simulink model "system1"  (R2020a)
settings: Solver=ode45  StartTime=0.0  StopTime=1  RelTol=1e-3
libraries: powerlib x28
settings Model: Creator=srish  LastModifiedBy=srishtik
settings DataIOCC: LimitDataPoints=on  SaveFormat=Array
settings OptimizationCC: BooleanDataType=off  LifeSpan=inf
settings DebuggingCC: ReadBeforeWriteMsg=DisableAll  WriteAfterWriteMsg=DisableAll  WriteAfterReadMsg=DisableAll  SaveWithParameterizedLinksMsg=none  UnderspecifiedInitializationDetection=Classic  MergeDetectMultiDrivingBlocksExec=none  MultiTaskDSMMsg=none  SFUnexpectedBacktrackingDiag=warning  SFNoUnconditionalDefaultTransitionDiag=warning  SFExecutionAtInitializationDiag=none  ArithmeticOperatorsInVariantConditions=warning
settings HardwareCC: ProdBitPerPointer=32  ProdBitPerSizeT=32  ProdBitPerPtrDiffT=32  ProdLargestAtomicFloat=None  ProdIntDivRoundTo=Undefined  ProdEndianess=Unspecified  ProdWordSize=32  ProdHWDeviceType=32-bit Generic  TargetUnknown=on
settings ModelReferenceCC: UpdateModelReferenceTargets=IfOutOfDate  PropagateSignalLabelsOutOfModel=off
settings SFSimCC: SFSimEcho=off  SimUseLocalCustomCode=off  CustomCodeUndefinedFunction=UseInterfaceOnly
settings RTWCC: RTWUseLocalCustomCode=off
settings CodeAppCC: StateflowObjectComments=on
settings GRTTargetCC: TargetLangStandard=C89/C90 (ANSI)
settings ConfigComp: CovMetricSettings=dw  CovHtmlReporting=on  CovSaveCumulativeToWorkspaceVar=on  CovSaveSingleToWorkspaceVar=on  CovExternalEMLEnable=off  CovSFcnEnable=off
settings SimscapeCC: SimscapeNormalizeSystem=off

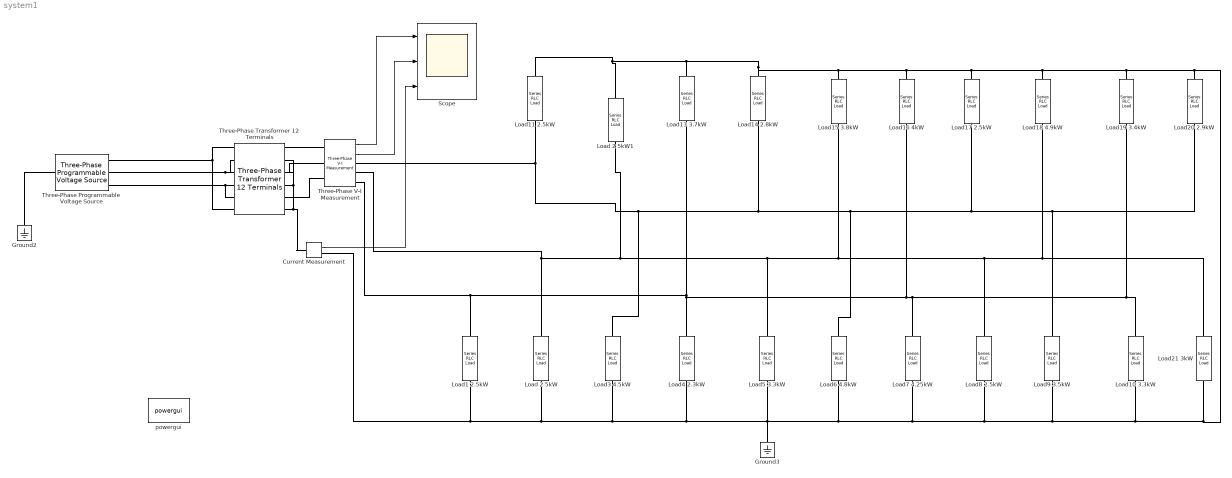
== system system1 ==
  " Load1 2.5kW" : powerlib/Elements/Series RLC Load  LConnTagsString=a  RConnTagsString=__new0  NominalVoltage=254  NominalFrequency=50  ActivePower=2500  InductivePower=1550  CapacitivePower=0  Setx0=off  InitialVoltage=0  SetiL0=off  InitialCurrent=0  Measurements=None  LoadType=constant Z
  " Load10 3.3kW " : powerlib/Elements/Series RLC Load  LConnTagsString=a  RConnTagsString=__new0  NominalVoltage=254  NominalFrequency=50  ActivePower=3300  InductivePower=2046  CapacitivePower=0  Setx0=off  InitialVoltage=0  SetiL0=off  InitialCurrent=0  Measurements=None  LoadType=constant Z
  " Load11 2.5kW" : powerlib/Elements/Series RLC Load  LConnTagsString=a  RConnTagsString=__new0  NominalVoltage=254  NominalFrequency=50  ActivePower=2500  InductivePower=1550  CapacitivePower=0  Setx0=off  InitialVoltage=0  SetiL0=off  InitialCurrent=0  Measurements=None  LoadType=constant Z
  " Load13 3.7kW" : powerlib/Elements/Series RLC Load  LConnTagsString=a  RConnTagsString=__new0  NominalVoltage=254  NominalFrequency=50  ActivePower=3700  InductivePower=2294  CapacitivePower=0  Setx0=off  InitialVoltage=0  SetiL0=off  InitialCurrent=0  Measurements=None  LoadType=constant Z
  " Load14 2.8kW" : powerlib/Elements/Series RLC Load  LConnTagsString=a  RConnTagsString=__new0  NominalVoltage=254  NominalFrequency=50  ActivePower=2800  InductivePower=1736  CapacitivePower=0  Setx0=off  InitialVoltage=0  SetiL0=off  InitialCurrent=0  Measurements=None  LoadType=constant Z
  " Load15 3.8kW" : powerlib/Elements/Series RLC Load  LConnTagsString=a  RConnTagsString=__new0  NominalVoltage=254  NominalFrequency=50  ActivePower=3800  InductivePower=2356  CapacitivePower=0  Setx0=off  InitialVoltage=0  SetiL0=off  InitialCurrent=0  Measurements=None  LoadType=constant Z
  " Load18 4.9kW" : powerlib/Elements/Series RLC Load  LConnTagsString=a  RConnTagsString=__new0  NominalVoltage=254  NominalFrequency=50  ActivePower=4900  InductivePower=3038  CapacitivePower=0  Setx0=off  InitialVoltage=0  SetiL0=off  InitialCurrent=0  Measurements=None  LoadType=constant Z
  " Load19 3.4kW" : powerlib/Elements/Series RLC Load  LConnTagsString=a  RConnTagsString=__new0  NominalVoltage=254  NominalFrequency=50  ActivePower=3400  InductivePower=2108  CapacitivePower=0  Setx0=off  InitialVoltage=0  SetiL0=off  InitialCurrent=0  Measurements=None  LoadType=constant Z
  " Load21 3kW" : powerlib/Elements/Series RLC Load  LConnTagsString=a  RConnTagsString=__new0  NominalVoltage=254  NominalFrequency=50  ActivePower=3000  InductivePower=1860  CapacitivePower=0  Setx0=off  InitialVoltage=0  SetiL0=off  InitialCurrent=0  Measurements=None  LoadType=constant Z
  " Load3 4.5kW" : powerlib/Elements/Series RLC Load  LConnTagsString=a  RConnTagsString=__new0  NominalVoltage=254  NominalFrequency=50  ActivePower=4500  InductivePower=2790  CapacitivePower=0  Setx0=off  InitialVoltage=0  SetiL0=off  InitialCurrent=0  Measurements=None  LoadType=constant Z
  " Load4 2.3kW " : powerlib/Elements/Series RLC Load  LConnTagsString=a  RConnTagsString=__new0  NominalVoltage=254  NominalFrequency=50  ActivePower=2300  InductivePower=1426  CapacitivePower=0  Setx0=off  InitialVoltage=0  SetiL0=off  InitialCurrent=0  Measurements=None  LoadType=constant Z
  " Load5 3.3kW" : powerlib/Elements/Series RLC Load  LConnTagsString=a  RConnTagsString=__new0  NominalVoltage=254  NominalFrequency=50  ActivePower=3300  InductivePower=2046  CapacitivePower=0  Setx0=off  InitialVoltage=0  SetiL0=off  InitialCurrent=0  Measurements=None  LoadType=constant Z
  " Load6 4.8kW" : powerlib/Elements/Series RLC Load  LConnTagsString=a  RConnTagsString=__new0  NominalVoltage=254  NominalFrequency=50  ActivePower=4800  InductivePower=2976  CapacitivePower=0  Setx0=off  InitialVoltage=0  SetiL0=off  InitialCurrent=0  Measurements=None  LoadType=constant Z
  " Load7 4.25kW" : powerlib/Elements/Series RLC Load  LConnTagsString=a  RConnTagsString=__new0  NominalVoltage=254  NominalFrequency=50  ActivePower=4250  InductivePower=2635  CapacitivePower=0  Setx0=off  InitialVoltage=0  SetiL0=off  InitialCurrent=0  Measurements=None  LoadType=constant Z
  " Load8 2.5kW" : powerlib/Elements/Series RLC Load  LConnTagsString=a  RConnTagsString=__new0  NominalVoltage=254  NominalFrequency=50  ActivePower=2500  InductivePower=1550  CapacitivePower=0  Setx0=off  InitialVoltage=0  SetiL0=off  InitialCurrent=0  Measurements=None  LoadType=constant Z
  " Load9 3.5kW" : powerlib/Elements/Series RLC Load  LConnTagsString=a  RConnTagsString=__new0  NominalVoltage=254  NominalFrequency=50  ActivePower=3500  InductivePower=2170  CapacitivePower=0  Setx0=off  InitialVoltage=0  SetiL0=off  InitialCurrent=0  Measurements=None  LoadType=constant Z
  Current Measurement : powerlib/Measurements/Current Measurement  PhasorSimulation=off  OutputType=Complex  PSBequivalent=0
  Ground2 : powerlib/Elements/Ground  LConnTagsString=a
  Ground3 : powerlib/Elements/Ground  LConnTagsString=a
  Load 2 5kW : powerlib/Elements/Series RLC Load  LConnTagsString=a  RConnTagsString=__new0  NominalVoltage=254  NominalFrequency=50  ActivePower=5000  InductivePower=3100  CapacitivePower=0  Setx0=off  InitialVoltage=0  SetiL0=off  InitialCurrent=0  Measurements=None  LoadType=constant Z
  Load 2 5kW1 : powerlib/Elements/Series RLC Load  LConnTagsString=a  RConnTagsString=__new0  NominalVoltage=254  NominalFrequency=50  ActivePower=5000  InductivePower=3100  CapacitivePower=0  Setx0=off  InitialVoltage=0  SetiL0=off  InitialCurrent=0  Measurements=None  LoadType=constant Z
  Load16 4kW : powerlib/Elements/Series RLC Load  LConnTagsString=a  RConnTagsString=__new0  NominalVoltage=254  NominalFrequency=50  ActivePower=4000  InductivePower=2480  CapacitivePower=0  Setx0=off  InitialVoltage=0  SetiL0=off  InitialCurrent=0  Measurements=None  LoadType=constant Z
  Load17 2.5kW : powerlib/Elements/Series RLC Load  LConnTagsString=a  RConnTagsString=__new0  NominalVoltage=254  NominalFrequency=50  ActivePower=2500  InductivePower=1550  CapacitivePower=0  Setx0=off  InitialVoltage=0  SetiL0=off  InitialCurrent=0  Measurements=None  LoadType=constant Z
  Load20 2.9kW : powerlib/Elements/Series RLC Load  LConnTagsString=a  RConnTagsString=__new0  NominalVoltage=254  NominalFrequency=50  ActivePower=2900  InductivePower=1798  CapacitivePower=0  Setx0=off  InitialVoltage=0  SetiL0=off  InitialCurrent=0  Measurements=None  LoadType=constant Z
  Scope : Scope  NumInputPorts=3
  Three-Phase Programmable Voltage Source : powerlib/Electrical Sources/Three-Phase Programmable Voltage Source  PositiveSequence="[6351  0 50]"  VariationEntity=None  VariationType=Table of time-amplitude pairs  VariationTypeAlt=Step  VariationStep=0.5  VariationRate=10  VariationMagnitude=0.3  VariationFrequency=2  VariationTiming=[1 2]  VariationPhaseA=off  Amplitudes=[1 0.8 1.2 1.0]  TimeValues=[0 0.1 0.15 0.2]  HarmonicGeneration=off  HarmonicA=[3 0.2 -25 0]  HarmonicB=[2 0.15 35 2]  Timing="[0.05  3]"  BusType=swing  Pref=0  Qref=0  Qmin=-inf  Qmax=inf
  Three-Phase V-I Measurement : powerlib/Measurements/Three-Phase V-I Measurement  VoltageMeasurement=phase-to-ground  SetLabelV=off  LabelV=Vabc  Vpu=off  VpuLL=off  CurrentMeasurement=yes  SetLabelI=off  LabelI=Iabc  Ipu=off  Pbase=100e6  Vbase=500e3  OutputType=Complex  PhasorSimulation=off  PSBequivalent=0
  Three-Phase Transformer 12 Terminals : powerlib/Elements/Three-Phase Transformer 12 Terminals  RatedPower=[ 10e6 50 ]  Winding1="[ 6351 0.002  0.05 ]"  Winding2=[ 254 0.002 0.05]  RmXm=[ 200 200 ]
      settings: SourceProductBaseCode=PS
  powergui : powerlib/powergui  Priority=1  SimulationMode=Continuous  SampleTime=50e-6  frequency=60  Iterations=50  frequencyindice=50  Pbase=100e6  ErrMax=1e-4  UnitsV=kV  UnitsW=MW  buscounter=0  FunctionMessages=off  echomessages=off  EnableUseOfTLC=off  CurrentSourceSwitches=off  DisableSnubberDevices=off  DisableRonSwitches=off  DisableVfSwitches=off  DisplayEquations=off  AutomaticDiscreteSolvers=off  SolverType=Tustin  Interpol=off  ExternalGateDelay=off  methode=off  Ts=0  x0status=blocks  SPID=off  SwTol=0  HookPort=off  NonlinearTolerance=1e-4  nMaxIteration=100  ContinueOnMaxIteration=off  RestoreLinks=warning  ResistiveCurrentMeasurement=off  Frange=[0:2:500]  Ylog=off  Xlog=on  ShowGrid=off  save=off  variable=ZData  structure=0  ZoomFFT=off  StartTime=0.0  cycles=1  DisplayStyle=1  fundamental=60  FreqAxis=off  MaxFrequency=1000  frequencyindicesteady=1  RmsSteady=1  display=off
  wires:
  Three-Phase V-I Measurement/1 -> Scope/1
  Three-Phase V-I Measurement/2 -> Scope/2
  Current Measurement/1 -> Scope/3
  connections:
  Load 2 5kW/RConn1 -- " Load3 4.5kW"/RConn1 -- " Load4 2.3kW "/RConn1 -- " Load5 3.3kW"/RConn1 -- " Load6 4.8kW"/RConn1 -- " Load7 4.25kW"/RConn1 -- " Load8 2.5kW"/RConn1 -- " Load9 3.5kW"/RConn1 -- " Load10 3.3kW "/RConn1 -- " Load21 3kW"/RConn1 -- Load 2 5kW1/LConn1 -- " Load11 2.5kW"/LConn1 -- " Load13 3.7kW"/LConn1 -- " Load14 2.8kW"/LConn1 -- " Load15 3.8kW"/LConn1 -- Load16 4kW/LConn1 -- Load17 2.5kW/LConn1 -- " Load18 4.9kW"/LConn1 -- " Load19 3.4kW"/LConn1 -- Load20 2.9kW/LConn1 -- Ground3/LConn1 -- Current Measurement/RConn1 -- " Load1 2.5kW"/RConn1
  Three-Phase Transformer 12 Terminals/RConn1 -- Three-Phase V-I Measurement/LConn1
  Three-Phase Transformer 12 Terminals/RConn3 -- Three-Phase V-I Measurement/LConn2
  Three-Phase Transformer 12 Terminals/RConn5 -- Three-Phase V-I Measurement/LConn3
  Three-Phase V-I Measurement/RConn3 -- Load16 4kW/RConn1 -- " Load19 3.4kW"/RConn1 -- " Load10 3.3kW "/LConn1 -- " Load7 4.25kW"/LConn1 -- " Load4 2.3kW "/LConn1 -- " Load13 3.7kW"/RConn1 -- " Load1 2.5kW"/LConn1
  Three-Phase V-I Measurement/RConn2 -- Load 2 5kW1/RConn1 -- " Load15 3.8kW"/RConn1 -- " Load18 4.9kW"/RConn1 -- " Load21 3kW"/LConn1 -- " Load8 2.5kW"/LConn1 -- " Load5 3.3kW"/LConn1 -- Load 2 5kW/LConn1
  Three-Phase V-I Measurement/RConn1 -- " Load3 4.5kW"/LConn1 -- " Load6 4.8kW"/LConn1 -- Load20 2.9kW/RConn1 -- " Load9 3.5kW"/LConn1 -- Load17 2.5kW/RConn1 -- " Load14 2.8kW"/RConn1 -- " Load11 2.5kW"/RConn1
  Three-Phase Programmable Voltage Source/LConn1 -- Ground2/LConn1
  Three-Phase Programmable Voltage Source/RConn1 -- Three-Phase Transformer 12 Terminals/LConn1 -- Three-Phase Transformer 12 Terminals/LConn6
  Three-Phase Transformer 12 Terminals/LConn3 -- Three-Phase Transformer 12 Terminals/LConn2 -- Three-Phase Programmable Voltage Source/RConn2
  Three-Phase Transformer 12 Terminals/LConn4 -- Three-Phase Transformer 12 Terminals/LConn5 -- Three-Phase Programmable Voltage Source/RConn3
  Current Measurement/LConn1 -- Three-Phase Transformer 12 Terminals/RConn2 -- Three-Phase Transformer 12 Terminals/RConn4 -- Three-Phase Transformer 12 Terminals/RConn6
